simulink model "stateSpace_design_bbsim_2022"  (R2022b)
settings: Solver=ode45  StartTime=0.0  StopTime=5  RelTol=1e-3
values from neighbouring files (symbols this model uses):
  Beq = 1.9610e-06    (= 1.961e-06)    [parameters.m]
  d = 1/sqrt(2)    [parameters.m]
  deg2V = 2.5/170    (= 0.0147058823529)    [parameters.m]
  Jeq = mot.J + mld.Jh/(gbox.N)^2    [parameters.m]
  K = lqr(sysG, Q, R)    [LQR_Bryson.m]    (also in LQR_design.m; stateSpace_Integral.m = K(2:end); stateSpace_Nominal.m = acker(A,B,eig); stateSpace_design.m = K(2:end))
  Ki = 0    [LQR_Bryson.m]    (also in LQR_design.m; stateSpace_Integral.m = K(1); stateSpace_Nominal.m; stateSpace_design.m = K(1))
  Nu = N(end)    [LQR_Bryson.m]    (also in stateSpace_Integral.m; stateSpace_Nominal.m; stateSpace_design.m)
  Nx = N(1:4)    [LQR_Bryson.m]    (also in stateSpace_Integral.m; stateSpace_Nominal.m; stateSpace_design.m)
  omega_c = 2*pi*50    (= 314.159265359)    [parameters.m]
  rads2rpm = 60/2/pi    (= 9.54929658551)    [parameters.m]
  rpm2rads = 2*pi/60    (= 0.10471975512)    [parameters.m]
  V2deg = 170/2.5    (= 68)    [parameters.m]
undefined symbols (not defined in the file or in its folder): DiscIntNeverNeededParam, drv, gbox, mld, mot, sens
libraries: hdlsllib x1
settings Model: Creator=gugli  LastModifiedBy=giuliapegoraro

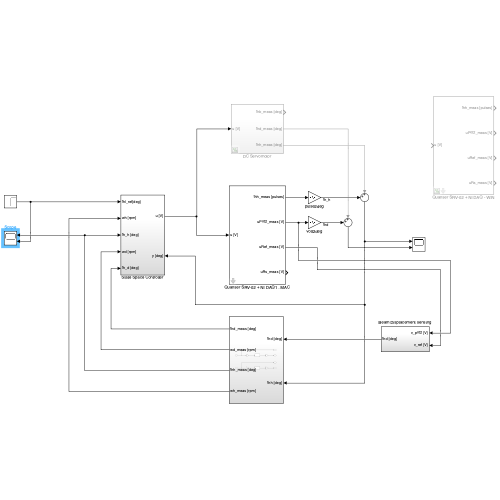
[thumbnail: Simulink's stored preview of the top-level diagram]
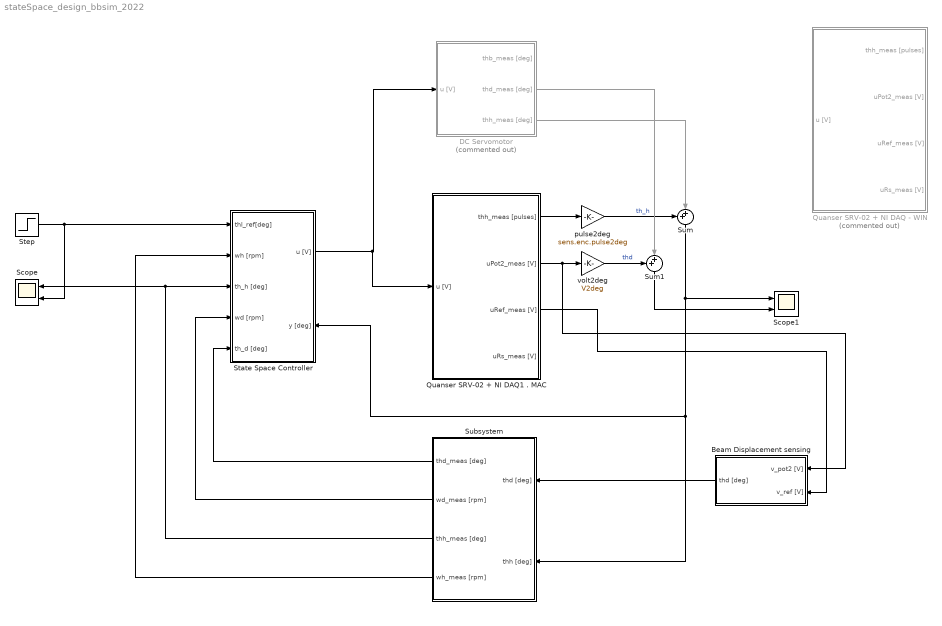
== system stateSpace_design_bbsim_2022 ==
  Beam Displacement sensing : Subsystem
  DC Servomotor : Subsystem  Commented=on
  Quanser SRV-02 + NI DAQ - WIN : Subsystem  Commented=on  mask(Quanser SRV-02 (with resonant load) + NI DAQ){Ts=0.001, fricType=Coulomb + viscous, lockShaft=off, beamInitPos=10}
      mask prompts: Ts "NI DAQ Sample Time:"; fricType "Friction model"; lockShaft "Lock motor shaft"; beamInitPos "Beam initial position [deg]:"
      mask help: Quanser SRV-02 (with resonant load) + NI DAQ model.
      mask init:
      | %%
      | % Riccardo Antonello (riccardo.antonello@unipd.it)
      | %
      | % April 28, 2020
      | %
      | % Dept. of Information Engineering, University of Padova
      | %
      | 
      | %%  Conversion gains
      | deg2rad = pi/180;                   %   [deg]   -> [rad]
      | rad2deg = 180/pi;                   %   [rad]   -> [deg]
      | 
      | 
      | %%  Sensors data
      | 
      | %   shunt resistor
      | sens.curr.Rs = 0.5;   
      | 
      | %   Hewlett-Packard HEDS-5540#A06 optical encoder
      | sens.enc.ppr = 500*4;                                                   %   pulses per rotation
      | sens.enc.pulse2deg = 360/sens.enc.ppr;                                  %   [pulses] -> [deg]
      | sens.enc.pulse2rad = 2*pi/sens.enc.ppr;                                 %   [pulses] -> [rad]
      | sens.enc.deg2pulse = sens.enc.ppr/360;                                  %   [deg] -> [pulses]
      | sens.enc.rad2pulse = sens.enc.ppr/2/pi;                                 %   [rad] -> [pulses]
      | 
      | %   potentiometer 2 (Spectrol 357-0-0-103) - installed on hub
      | sens.pot2.range.R      = 10e3;                                          %   ohmic value range 
      | sens.pot2.range.V      = 5;                                             %   voltage range
      | sens.pot2.range.th_deg = 340;                                           %   angle range [deg]
      | sens.pot2.range.th     = sens.pot2.range.th_deg * deg2rad;              %   angle range [rad]                           
      | sens.pot2.deg2V        = sens.pot2.range.V / sens.pot2.range.th_deg;    %   sensitivity [V/deg]
      | sens.pot2.rad2V        = sens.pot2.range.V / sens.pot2.range.th;        %   sensitivity [V/rad]
      | sens.pot2.V2deg        = 1/sens.pot2.deg2V;                             %   conversion gain [V] -> [deg]
      | sens.pot2.V2rad        = 1/sens.pot2.rad2V;                             %   conversion gain [V] -> [rad]
      | sens.pot2.noise.var    = 3.5e-7;                                        %   out noise variance [V^2]
      | 
      | 
      | %%  Data acquisition board (daq) data
      | 
      | %   NI PCI-6221 DAC data
      | daq.dac.bits = 16;                                  %   resolution (bits)
      | daq.dac.fs   = 10;                                  %   full scale 
      | daq.dac.q    = 2*daq.dac.fs/(2^daq.dac.bits-1);     %	quantization
      | 
      | %   NI PCI-6221 ADC data
      | daq.adc.bits = 16;                                  %   resolution (bits)
      | daq.adc.fs   = 10;                                  %   full scale (as set in SLDRT Analog Input block)
      | daq.adc.q    = 2*daq.adc.fs/(2^daq.adc.bits-1);     %   quantization   
      | 
      | 
      | %%  Set beam initial position
      | % SRV02Handle = find_system(gcb, ...
      | %     'LookUnderMasks', 'on', ...
      | %     'FindAll', 'on', ...
      | %     'FollowLinks', 'on', ...
      | %     'SearchDepth', '1', ...
      | %     'BlockType', 'ModelReference', ...
      | %     'Name', 'Quanser SRV-02');
      | %
      | % %get_param(SRV02Handle, 'InstanceParameters')
      | % InstanceParams = get_param(SRV02Handle, 'InstanceParameters');
      | % for k = 1:length(InstanceParams)
      | %     if strcmp(InstanceParams(k).Name, 'thb0')
      | %         if lockShaft
      | %             InstanceParams(k).Value = sprintf('%f', beamInitPos);
      | %         else
      | %             InstanceParams(k).Value = sprintf('%f', 0);    
      | %         end
      | %         set_param(SRV02Handle, 'InstanceParameters', InstanceParams);
      | %         break;
      | %     end
      | % end
      | 
      | if lockShaft
      |     thb0 = beamInitPos;
      | else
      |     thb0 = 0;    
      | end
      | 
      | 
      | %%  Mask initialization
      | if lockShaft
      |     
      |     %   find Inport handle
      |     InPortHandle = find_system(gcb, ...
      |         'LookUnderMasks', 'on', ...
      |         'FindAll', 'on', ...
      |         'FollowLinks', 'on', ...
      |         'SearchDepth', '1', ...
      |         'BlockType', 'Inport', ...
      |         'Name', 'u [V]');
      |     
      |     if ~isempty(InPortHandle)
      |     
      |         %   find DAC handle
      |         DACHandle = find_system(gcb, ...
      |             'LookUnderMasks', 'on', ...
      |             'FindAll', 'on', ...
      |             'FollowLinks', 'on', ...
      |             'SearchDepth', '1', ...
      |             'BlockType', 'SubSystem', ...
      |             'Name', 'DAC');  
      | 
      |         %   remove Inport output connection   
      |         InportConn = get_param(InPortHandle, 'PortConnectivity');
      |         delete_line(gcb, InportConn.Position);
      | 
      |         %   remove Inport block
      |         delete_block(InPortHandle);
      | 
      |         %   add Constant block
      |         ConstantHandle = add_block( ...
      |             'simulink/Sources/Constant', [gcb, '/u [V]'], ...
      |             'Position', [20   -37    50   -23], ...
      |             'Value', '0');
      | 
      |         %   connect Constant to DAC block
      |         DACPortHandles = get_param(DACHandle, 'PortHandles');
      |         ConstantPortHandles = get_param(ConstantHandle, 'PortHandles');
      |         add_line(gcb, ConstantPortHandles.Outport(1), DACPortHandles.Inport(1));
      |     
      |     end
      |     
      | else
      |     
      |     %   find Constant handle
      |     ConstantHandle = find_system(gcb, ...
      |         'LookUnderMasks', 'on', ...
      |         'FindAll', 'on', ...
      |         'FollowLinks', 'on', ...
      |         'SearchDepth', '1', ...
      |         'BlockType', 'Constant', ...
      |         'Name', 'u [V]');
      |     
      |     if ~isempty(ConstantHandle)
      |     
      |         %   find DAC handle
      |         DACHandle = find_system(gcb, ...
      |             'LookUnderMasks', 'on', ...
      |             'FindAll', 'on', ...
      |             'FollowLinks', 'on', ...
      |             'SearchDepth', '1', ...
      |             'BlockType', 'SubSystem', ...
      |             'Name', 'DAC');  
      |  
      |         %   remove Constant output connection   
      |         ConstantConn = get_param(ConstantHandle, 'PortConnectivity');
      |         delete_line(gcb, ConstantConn.Position);
      | 
      |         %   remove Inport block
      |         delete_block(ConstantHandle);   
      | 
      |         %   add Inport block
      |         InportHandle = add_block( ...
      |             'simulink/Sources/In1', [gcb, '/u [V]'], ...
      |             'Position', [20   -37    50   -23], ...
      |             'Port', '1');
      | 
      |         %   connect Constant to DAC block
      |         DACPortHandles = get_param(DACHandle, 'PortHandles');
      |         InportPortHandles = get_param(InportHandle, 'PortHandles');
      |         add_line(gcb, InportPortHandles.Outport(1), DACPortHandles.Inport(1));
      |     
      |      end
      |     
      | end
      mask Help:
      | Riccardo Antonello (antonello@dei.unipd.it)
      | 
      | April 28, 2020
      | 
      | Dept. of Information Engineering, University of Padova
      mask TypeOptions fricType: Coulomb + viscous | Karnopp
      mask Callback lockShaft:
      | %   get status of check box
      | lockShaft = get_param(gcb, 'lockShaft');
      | 
      | %   get current value of MaskVisibilities property
      | maskVisibilities = get_param(gcb, 'MaskVisibilities');
      | 
      | %   set visibility of the dialog box element
      | if strcmp(lockShaft, 'on')
      |     maskVisibilities{4} = 'on';
      | else
      |     maskVisibilities{4} = 'off';
      | end
      | 
      | % Set the 'MaskVisibilities' property for each parameter in mask
      | set_param( gcb, 'MaskVisibilities', maskVisibilities);
  Quanser SRV-02 + NI DAQ1 . MAC : Subsystem  mask(Quanser SRV-02 (with resonant load) + NI DAQ){Ts=0.001, fricType=Coulomb + viscous, lockShaft=off, beamInitPos=10}
      mask prompts: Ts "NI DAQ Sample Time:"; fricType "Friction model"; lockShaft "Lock motor shaft"; beamInitPos "Beam initial position [deg]:"
      mask help: Quanser SRV-02 (with resonant load) + NI DAQ model.
      mask init: same as stateSpace_design_bbsim_2022/Quanser SRV-02 + NI DAQ - WIN
      mask Help:
      | Riccardo Antonello (antonello@dei.unipd.it)
      | 
      | April 28, 2020
      | 
      | Dept. of Information Engineering, University of Padova
      mask TypeOptions fricType: Coulomb + viscous | Karnopp
      mask Callback lockShaft:
      | %   get status of check box
      | lockShaft = get_param(gcb, 'lockShaft');
      | 
      | %   get current value of MaskVisibilities property
      | maskVisibilities = get_param(gcb, 'MaskVisibilities');
      | 
      | %   set visibility of the dialog box element
      | if strcmp(lockShaft, 'on')
      |     maskVisibilities{4} = 'on';
      | else
      |     maskVisibilities{4} = 'off';
      | end
      | 
      | % Set the 'MaskVisibilities' property for each parameter in mask
      | set_param( gcb, 'MaskVisibilities', maskVisibilities);
  Scope : Scope  NumInputPorts=2
  Scope1 : Scope  NumInputPorts=2
  State Space Controller : Subsystem
      settings: PortSchema="{\"entries\":[{\"content\":{\"sides\":[{\"content\":{\"connectorIds\":[\"In1\",\"In2\",\"In3\",\"In4\",\"In5\"]},\"type\":\"ConnectorPlacement.EquallySpacedRectSide\",\"uuid\":\"18355374-ba4e-4826-b39c-e1fec12a3224\"},{\"content\":{\"connectorIds\":[\"Out1\",\"In6\"],\"side\":\"RIGHT\"},\"type\":\"ConnectorPlacement.EquallySpacedRectSide\",\"uuid\":\"1b1017b5-1e71-4f75-9751-b5be90c6ae70\"},{\"content\":{\"connectorIds\":[],\"side\":\"TOP\"},\"type\":\"ConnectorPlacement.EquallySpacedRectSide\",\"uuid\":\"216eee75-1744-4a6a-833a-20d97cc02b89\"}]},\"type\":\"ConnectorPlacement.EquallySpacedConnector\",\"uuid\":\"af6359b3-3eb7-4cad-ada4-005509c30a45\"}],\"packageUris\":[\"http://schema.mathworks.com/mf0/Connector/R2020b\"],\"version\":\"1.0\"}"
  Step : Step  After=50
  Subsystem : Subsystem
  Sum : Sum  Inputs=++|
  Sum1 : Sum  Inputs=++|
  pulse2deg : Gain  Gain=sens.enc.pulse2deg
  volt2deg : Gain  Gain=V2deg
  wires:
  Step/1 -> Scope/2, State Space Controller/1(thl_ref[deg])
  pulse2deg/1 -> Sum/1  "th_h"
  DC Servomotor/3(thh_meas [deg]) -> Sum/2
  Quanser SRV-02 + NI DAQ1 . MAC/1(thh_meas [pulses]) -> pulse2deg/1
  State Space Controller/1(u [V]) -> Quanser SRV-02 + NI DAQ1 . MAC/1(u [V]), DC Servomotor/1(u [V])
  Quanser SRV-02 + NI DAQ1 . MAC/2(uPot2_meas [V]) -> Beam Displacement sensing/1(v_pot2 [V]), volt2deg/1
  Subsystem/1(thd_meas [deg]) -> State Space Controller/5(th_d [deg])
  Subsystem/2(wd_meas [rpm]) -> State Space Controller/4(wd [rpm])
  Subsystem/3(thh_meas [deg]) -> Scope/1, State Space Controller/3(th_h [deg])
  Subsystem/4(wh_meas [rpm]) -> State Space Controller/2(wh [rpm])
  Sum1/1 -> Scope1/2
  volt2deg/1 -> Sum1/1  "thd"
  DC Servomotor/2(thd_meas [deg]) -> Sum1/2
  Sum/1 -> State Space Controller/6(y [deg]), Subsystem/2(thh [deg]), Scope1/1
  Quanser SRV-02 + NI DAQ1 . MAC/3(uRef_meas [V]) -> Beam Displacement sensing/2(v_ref [V])
  Beam Displacement sensing/1(thd [deg]) -> Subsystem/1(thd [deg])

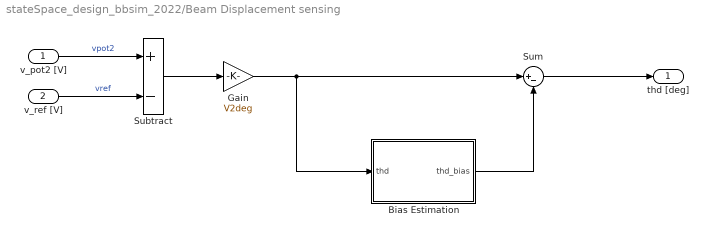
== system stateSpace_design_bbsim_2022/Beam Displacement sensing ==
  v_pot2 [V] : Inport
  v_ref [V] : Inport  Port=2
  Bias Estimation : Subsystem
  Gain : Gain  Gain=V2deg
  Subtract : Sum  Inputs=+-
  Sum : Sum  Inputs=|+-
  thd [deg] : Outport
  wires:
  v_ref [V]/1 -> Subtract/2  "vref"
  v_pot2 [V]/1 -> Subtract/1  "vpot2"
  Subtract/1 -> Gain/1
  Gain/1 -> Bias Estimation/1(thd), Sum/1
  Sum/1 -> thd [deg]/1
  Bias Estimation/1(thd_bias) -> Sum/2

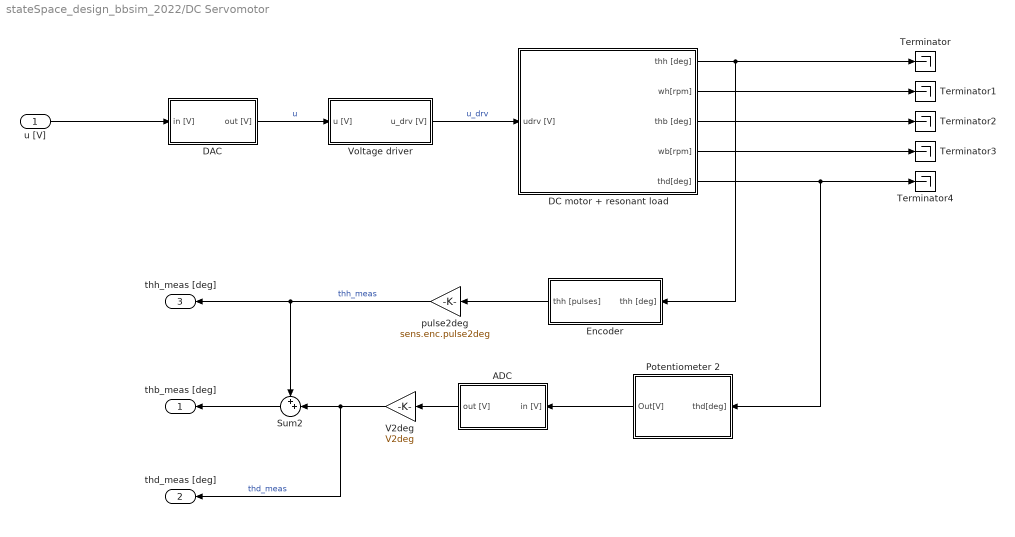
== system stateSpace_design_bbsim_2022/DC Servomotor ==
  u [V] : Inport
  ADC : Subsystem
  DAC : Subsystem
  DC motor + resonant load : Subsystem
  Encoder : Subsystem
  Potentiometer 2 : Subsystem
  Sum2 : Sum  Inputs=++|
  Terminator{,1..4} (5 alike) : Terminator
  V2deg : Gain  Gain=V2deg
  Voltage driver : Subsystem
  pulse2deg : Gain  Gain=sens.enc.pulse2deg
  thb_meas [deg] : Outport
  thd_meas [deg] : Outport  Port=2
  thh_meas [deg] : Outport  Port=3
  wires:
  Encoder/1(thh [pulses]) -> pulse2deg/1
  DAC/1(out [V]) -> Voltage driver/1(u [V])  "u"
  pulse2deg/1 -> thh_meas [deg]/1, Sum2/1  "thh_meas"
  u [V]/1 -> DAC/1(in [V])
  DC motor + resonant load/1(thh [deg]) -> Encoder/1(thh [deg]), Terminator/1
  DC motor + resonant load/2(wh[rpm]) -> Terminator1/1
  Voltage driver/1(u_drv [V]) -> DC motor + resonant load/1(udrv [V])  "u_drv"
  DC motor + resonant load/3(thb [deg]) -> Terminator2/1
  DC motor + resonant load/4(wb[rpm]) -> Terminator3/1
  DC motor + resonant load/5(thd[deg]) -> Potentiometer 2/1(thd[deg]), Terminator4/1
  Potentiometer 2/1(Out[V]) -> ADC/1(in [V])
  ADC/1(out [V]) -> V2deg/1
  V2deg/1 -> thd_meas [deg]/1, Sum2/2  "thd_meas"
  Sum2/1 -> thb_meas [deg]/1

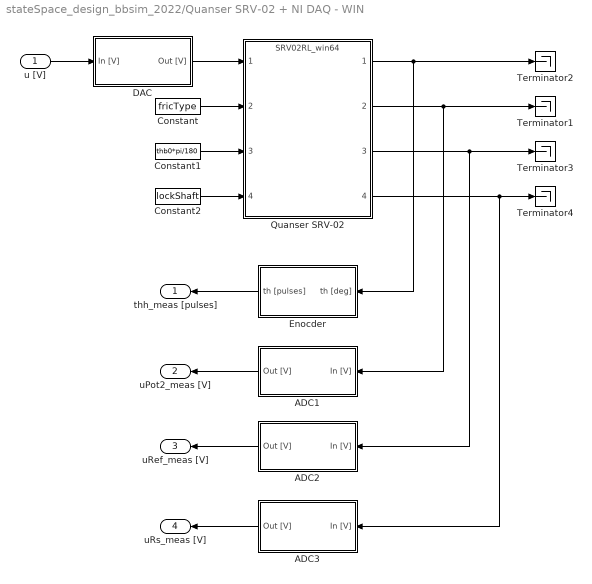
== system stateSpace_design_bbsim_2022/Quanser SRV-02 + NI DAQ - WIN ==
  u [V] : Inport
  ADC1 : Subsystem
  ADC2 : Subsystem
  ADC3 : Subsystem
  Constant : Constant  Value=fricType
  Constant1 : Constant  Value=thb0*pi/180  SampleTime=Inf
  Constant2 : Constant  Value=lockShaft  SampleTime=Inf
  DAC : Subsystem
  Enocder : Subsystem
  Quanser SRV-02 : ModelReference  ModelNameDialog=SRV02RL_win64.slxp  ModelReferenceVersion=1.76  CopyOfModelProtected=on
  Terminator{1..4} (4 alike) : Terminator
  thh_meas [pulses] : Outport
  uPot2_meas [V] : Outport  Port=2
  uRef_meas [V] : Outport  Port=3
  uRs_meas [V] : Outport  Port=4
  wires:
  u [V]/1 -> DAC/1(In [V])
  ADC2/1(Out [V]) -> uRef_meas [V]/1
  Quanser SRV-02/4 -> Terminator4/1, ADC3/1(In [V])
  Constant2/1 -> Quanser SRV-02/4
  Constant1/1 -> Quanser SRV-02/3
  ADC1/1(Out [V]) -> uPot2_meas [V]/1
  Quanser SRV-02/3 -> Terminator3/1, ADC2/1(In [V])
  Constant/1 -> Quanser SRV-02/2
  Quanser SRV-02/1 -> Enocder/1(th [deg]), Terminator2/1
  Quanser SRV-02/2 -> Terminator1/1, ADC1/1(In [V])
  DAC/1(Out [V]) -> Quanser SRV-02/1
  ADC3/1(Out [V]) -> uRs_meas [V]/1
  Enocder/1(th [pulses]) -> thh_meas [pulses]/1

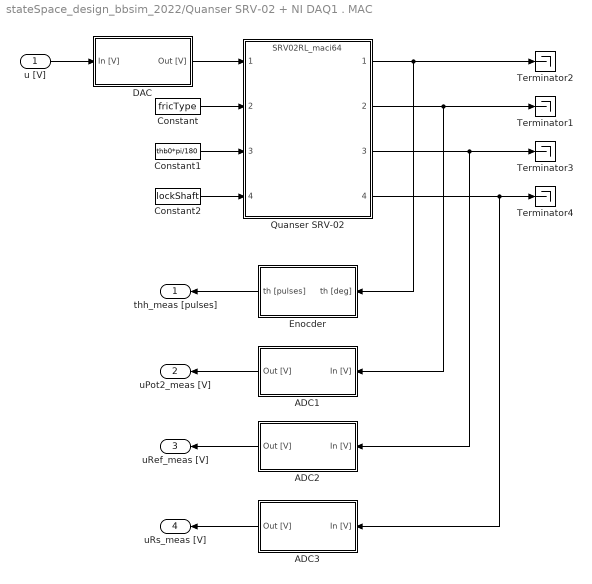
== system stateSpace_design_bbsim_2022/Quanser SRV-02 + NI DAQ1 . MAC ==
  u [V] : Inport
  ADC1 : Subsystem
  ADC2 : Subsystem
  ADC3 : Subsystem
  Constant : Constant  Value=fricType
  Constant1 : Constant  Value=thb0*pi/180  SampleTime=Inf
  Constant2 : Constant  Value=lockShaft  SampleTime=Inf
  DAC : Subsystem
  Enocder : Subsystem
  Quanser SRV-02 : ModelReference  ModelNameDialog=SRV02RL_maci64.slxp  ModelReferenceVersion=1.76  CopyOfModelProtected=on
  Terminator{1..4} (4 alike) : Terminator
  thh_meas [pulses] : Outport
  uPot2_meas [V] : Outport  Port=2
  uRef_meas [V] : Outport  Port=3
  uRs_meas [V] : Outport  Port=4
  wires:
  Enocder/1(th [pulses]) -> thh_meas [pulses]/1
  ADC3/1(Out [V]) -> uRs_meas [V]/1
  DAC/1(Out [V]) -> Quanser SRV-02/1
  Quanser SRV-02/2 -> ADC1/1(In [V]), Terminator1/1
  Quanser SRV-02/1 -> Terminator2/1, Enocder/1(th [deg])
  Constant/1 -> Quanser SRV-02/2
  Quanser SRV-02/3 -> ADC2/1(In [V]), Terminator3/1
  ADC1/1(Out [V]) -> uPot2_meas [V]/1
  Constant1/1 -> Quanser SRV-02/3
  Constant2/1 -> Quanser SRV-02/4
  u [V]/1 -> DAC/1(In [V])
  Quanser SRV-02/4 -> ADC3/1(In [V]), Terminator4/1
  ADC2/1(Out [V]) -> uRef_meas [V]/1

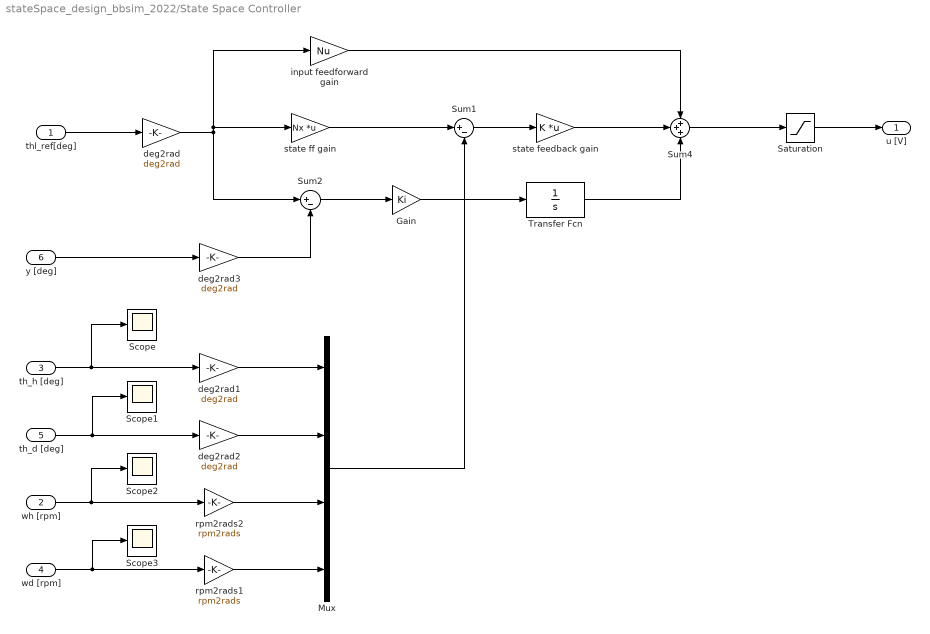
== system stateSpace_design_bbsim_2022/State Space Controller ==
  thl_ref[deg] : Inport
  wh [rpm] : Inport  Port=2
  th_h [deg] : Inport  Port=3
  wd [rpm] : Inport  Port=4
  th_d [deg] : Inport  Port=5
  y [deg] : Inport  Port=6
  " Saturation" : Saturate  UpperLimit=12  LowerLimit=-12
  Gain : Gain  Gain=Ki
  Mux : Mux
  Scope{,1..3} (4 alike) : Scope
  Sum1 : Sum  Inputs=|+-
  Sum2 : Sum  Inputs=|+-
  Sum4 : Sum  Inputs=+++
  Transfer Fcn : TransferFcn  Numerator=1  Denominator=[1 0]
  deg2rad{,1..3} (4 alike) : Gain  Gain=deg2rad
  input feedforward gain : Gain  Gain=Nu
  rpm2rads1 : Gain  Gain=rpm2rads
  rpm2rads2 : Gain  Gain=rpm2rads
  state feedback gain : Gain  Gain=K  Multiplication=Matrix(K*u) (u vector)
  state ff gain : Gain  Gain=Nx  Multiplication=Matrix(K*u) (u vector)
  u [V] : Outport
  wires:
  thl_ref[deg]/1 -> deg2rad/1
  deg2rad/1 -> state ff gain/1, input feedforward gain/1, Sum2/1
  state ff gain/1 -> Sum1/1
  Sum1/1 -> state feedback gain/1
  state feedback gain/1 -> Sum4/2
  input feedforward gain/1 -> Sum4/1
  Sum4/1 -> " Saturation"/1
  " Saturation"/1 -> u [V]/1
  Mux/1 -> Sum1/2
  deg2rad1/1 -> Mux/1
  th_h [deg]/1 -> Scope/1, deg2rad1/1
  wd [rpm]/1 -> Scope3/1, rpm2rads1/1
  rpm2rads1/1 -> Mux/4
  Gain/1 -> Transfer Fcn/1
  Transfer Fcn/1 -> Sum4/3
  y [deg]/1 -> deg2rad3/1
  deg2rad3/1 -> Sum2/2
  Sum2/1 -> Gain/1
  rpm2rads2/1 -> Mux/3
  deg2rad2/1 -> Mux/2
  th_d [deg]/1 -> Scope1/1, deg2rad2/1
  wh [rpm]/1 -> Scope2/1, rpm2rads2/1

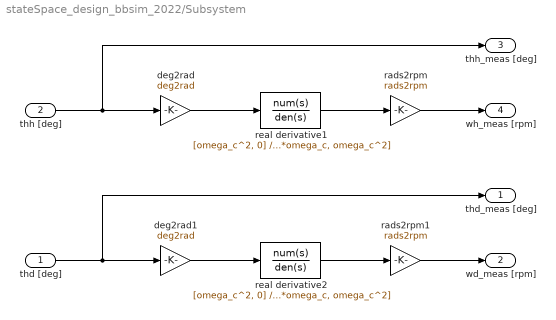
== system stateSpace_design_bbsim_2022/Subsystem ==
  thd [deg] : Inport
  thh [deg] : Inport  Port=2
  deg2rad : Gain  Gain=deg2rad
  deg2rad1 : Gain  Gain=deg2rad
  rads2rpm : Gain  Gain=rads2rpm
  rads2rpm1 : Gain  Gain=rads2rpm
  real derivative1 : TransferFcn  Numerator=[omega_c^2, 0]  Denominator=[1, 2*d*omega_c, omega_c^2]
  real derivative2 : TransferFcn  Numerator=[omega_c^2, 0]  Denominator=[1, 2*d*omega_c, omega_c^2]
  thd_meas [deg] : Outport
  wd_meas [rpm] : Outport  Port=2
  thh_meas [deg] : Outport  Port=3
  wh_meas [rpm] : Outport  Port=4
  wires:
  deg2rad/1 -> real derivative1/1
  thh [deg]/1 -> thh_meas [deg]/1, deg2rad/1
  real derivative1/1 -> rads2rpm/1
  rads2rpm/1 -> wh_meas [rpm]/1
  rads2rpm1/1 -> wd_meas [rpm]/1
  thd [deg]/1 -> thd_meas [deg]/1, deg2rad1/1
  deg2rad1/1 -> real derivative2/1
  real derivative2/1 -> rads2rpm1/1

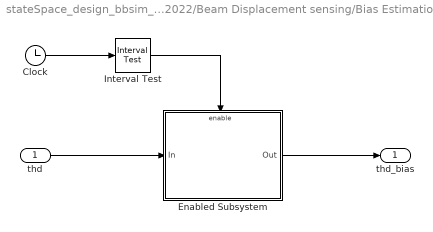
== system stateSpace_design_bbsim_2022/Beam Displacement sensing/Bias Estimation ==
  thd : Inport
  Clock : Clock
  Enabled Subsystem : Subsystem  TreatAsAtomicUnit=on
  Interval Test : hdlsllib/Logic and Bit Operations/Interval Test  IntervalClosedRight=on  uplimit=0.5  IntervalClosedLeft=on  lowlimit=-0.5  OutDataTypeStr=boolean
  thd_bias : Outport
  wires:
  thd/1 -> Enabled Subsystem/1(In)
  Enabled Subsystem/1(Out) -> thd_bias/1
  Clock/1 -> Interval Test/1
  Interval Test/1 -> Enabled Subsystem/Enable

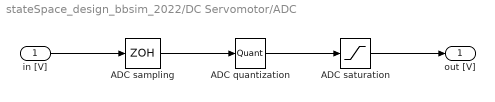
== system stateSpace_design_bbsim_2022/DC Servomotor/ADC ==
  in [V] : Inport
  ADC quantization : Quantizer  QuantizationInterval=daq.adc.q
  ADC sampling : ZeroOrderHold  SampleTime=0.001
  ADC saturation : Saturate  UpperLimit=10  LowerLimit=-10
  out [V] : Outport
  wires:
  ADC saturation/1 -> out [V]/1
  ADC quantization/1 -> ADC saturation/1
  in [V]/1 -> ADC sampling/1
  ADC sampling/1 -> ADC quantization/1

== system stateSpace_design_bbsim_2022/DC Servomotor/DAC ==
  in [V] : Inport
  Quantizer : Quantizer  QuantizationInterval=daq.dac.q
  Saturation : Saturate  UpperLimit=10  LowerLimit=-10
  Zero-Order Hold : ZeroOrderHold  SampleTime=0.001
  out [V] : Outport
  wires:
  Saturation/1 -> out [V]/1
  Quantizer/1 -> Saturation/1
  in [V]/1 -> Zero-Order Hold/1
  Zero-Order Hold/1 -> Quantizer/1

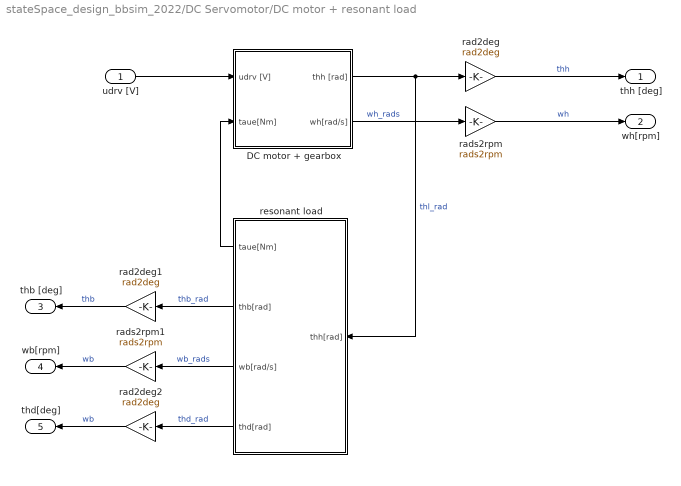
== system stateSpace_design_bbsim_2022/DC Servomotor/DC motor + resonant load ==
  udrv [V] : Inport
  DC motor + gearbox : Subsystem
  rad2deg : Gain  Gain=rad2deg
  rad2deg1 : Gain  Gain=rad2deg
  rad2deg2 : Gain  Gain=rad2deg
  rads2rpm : Gain  Gain=rads2rpm
  rads2rpm1 : Gain  Gain=rads2rpm
  resonant load : Subsystem
  thh [deg] : Outport
  wh[rpm] : Outport  Port=2
  thb [deg] : Outport  Port=3
  wb[rpm] : Outport  Port=4
  thd[deg] : Outport  Port=5
  wires:
  DC motor + gearbox/1(thh [rad]) -> resonant load/1(thh[rad]), rad2deg/1  "thl_rad"
  rad2deg2/1 -> thd[deg]/1  "wb"
  resonant load/1(taue[Nm]) -> DC motor + gearbox/2(taue[Nm])
  DC motor + gearbox/2(wh[rad/s]) -> rads2rpm/1  "wh_rads"
  rad2deg/1 -> thh [deg]/1  "thh"
  resonant load/4(thd[rad]) -> rad2deg2/1  "thd_rad"
  rads2rpm/1 -> wh[rpm]/1  "wh"
  udrv [V]/1 -> DC motor + gearbox/1(udrv [V])
  resonant load/2(thb[rad]) -> rad2deg1/1  "thb_rad"
  resonant load/3(wb[rad/s]) -> rads2rpm1/1  "wb_rads"
  rads2rpm1/1 -> wb[rpm]/1  "wb"
  rad2deg1/1 -> thb [deg]/1  "thb"

== system stateSpace_design_bbsim_2022/DC Servomotor/Encoder ==
  thh [deg] : Inport
  Gain : Gain  Gain=1/sens.enc.pulse2deg
  Quantizer : Quantizer  QuantizationInterval=sens.enc.pulse2deg
  Zero-Order Hold : ZeroOrderHold  SampleTime=0.001
  thh [pulses] : Outport
  wires:
  Zero-Order Hold/1 -> Quantizer/1
  thh [deg]/1 -> Zero-Order Hold/1
  Quantizer/1 -> Gain/1
  Gain/1 -> thh [pulses]/1

== system stateSpace_design_bbsim_2022/DC Servomotor/Potentiometer 2 ==
  thd[deg] : Inport
  Sum2 : Sum  Inputs=++|
  deg2V : Gain  Gain=deg2V
  sensor output noise [V] : RandomNumber  Variance=3.5*10^[-7]  SampleTime=0.001
  Out[V] : Outport
  wires:
  Sum2/1 -> Out[V]/1
  sensor output noise [V]/1 -> Sum2/1
  deg2V/1 -> Sum2/2  "thl_meas"
  thd[deg]/1 -> deg2V/1

== system stateSpace_design_bbsim_2022/DC Servomotor/Voltage driver ==
  u [V] : Inport
  Saturation : Saturate  UpperLimit=12  LowerLimit=-12
  Transfer Fcn : TransferFcn  Numerator=[drv.dcgain]  Denominator=[drv.Tc 1]
  u_drv [V] : Outport
  wires:
  Saturation/1 -> u_drv [V]/1
  Transfer Fcn/1 -> Saturation/1
  u [V]/1 -> Transfer Fcn/1

== system stateSpace_design_bbsim_2022/Quanser SRV-02 + NI DAQ - WIN/ADC1 ==
  In [V] : Inport
  ADC quantization : Quantizer  QuantizationInterval=daq.adc.q
  ADC sampling : ZeroOrderHold  SampleTime=Ts
  ADC saturation : Saturate  UpperLimit=daq.adc.fs  LowerLimit=-daq.adc.fs
  Out [V] : Outport
  wires:
  ADC quantization/1 -> ADC saturation/1
  In [V]/1 -> ADC sampling/1
  ADC sampling/1 -> ADC quantization/1
  ADC saturation/1 -> Out [V]/1

== system stateSpace_design_bbsim_2022/Quanser SRV-02 + NI DAQ - WIN/ADC2 ==
  In [V] : Inport
  ADC quantization : Quantizer  QuantizationInterval=daq.adc.q
  ADC sampling : ZeroOrderHold  SampleTime=Ts
  ADC saturation : Saturate  UpperLimit=daq.adc.fs  LowerLimit=-daq.adc.fs
  Out [V] : Outport
  wires:
  ADC saturation/1 -> Out [V]/1
  ADC sampling/1 -> ADC quantization/1
  In [V]/1 -> ADC sampling/1
  ADC quantization/1 -> ADC saturation/1

== system stateSpace_design_bbsim_2022/Quanser SRV-02 + NI DAQ - WIN/ADC3 ==
  In [V] : Inport
  Quantizer : Quantizer  QuantizationInterval=daq.adc.q
  Saturation : Saturate  UpperLimit=daq.adc.fs  LowerLimit=-daq.adc.fs
  Zero-Order Hold : ZeroOrderHold  SampleTime=Ts
  Out [V] : Outport
  wires:
  Zero-Order Hold/1 -> Quantizer/1
  Quantizer/1 -> Saturation/1
  In [V]/1 -> Zero-Order Hold/1
  Saturation/1 -> Out [V]/1

== system stateSpace_design_bbsim_2022/Quanser SRV-02 + NI DAQ - WIN/DAC ==
  In [V] : Inport
  Quantizer : Quantizer  QuantizationInterval=daq.dac.q
  Saturation : Saturate  UpperLimit=daq.dac.fs  LowerLimit=-daq.dac.fs
  Zero-Order Hold : ZeroOrderHold  SampleTime=Ts
  Out [V] : Outport
  wires:
  Saturation/1 -> Out [V]/1
  Zero-Order Hold/1 -> Quantizer/1
  In [V]/1 -> Zero-Order Hold/1
  Quantizer/1 -> Saturation/1

== system stateSpace_design_bbsim_2022/Quanser SRV-02 + NI DAQ - WIN/Enocder ==
  th [deg] : Inport
  Quantizer : Quantizer  QuantizationInterval=sens.enc.pulse2deg
  Zero-Order Hold : ZeroOrderHold  SampleTime=Ts
  deg2pulse : Gain  Gain=sens.enc.deg2pulse
  th [pulses] : Outport
  wires:
  deg2pulse/1 -> th [pulses]/1
  Zero-Order Hold/1 -> Quantizer/1
  th [deg]/1 -> Zero-Order Hold/1
  Quantizer/1 -> deg2pulse/1

== system stateSpace_design_bbsim_2022/Quanser SRV-02 + NI DAQ1 . MAC/ADC1 ==
  In [V] : Inport
  ADC quantization : Quantizer  QuantizationInterval=daq.adc.q
  ADC sampling : ZeroOrderHold  SampleTime=Ts
  ADC saturation : Saturate  UpperLimit=daq.adc.fs  LowerLimit=-daq.adc.fs
  Out [V] : Outport
  wires:
  ADC saturation/1 -> Out [V]/1
  ADC sampling/1 -> ADC quantization/1
  In [V]/1 -> ADC sampling/1
  ADC quantization/1 -> ADC saturation/1

== system stateSpace_design_bbsim_2022/Quanser SRV-02 + NI DAQ1 . MAC/ADC2 ==
  In [V] : Inport
  ADC quantization : Quantizer  QuantizationInterval=daq.adc.q
  ADC sampling : ZeroOrderHold  SampleTime=Ts
  ADC saturation : Saturate  UpperLimit=daq.adc.fs  LowerLimit=-daq.adc.fs
  Out [V] : Outport
  wires:
  ADC quantization/1 -> ADC saturation/1
  In [V]/1 -> ADC sampling/1
  ADC sampling/1 -> ADC quantization/1
  ADC saturation/1 -> Out [V]/1

== system stateSpace_design_bbsim_2022/Quanser SRV-02 + NI DAQ1 . MAC/ADC3 ==
  In [V] : Inport
  Quantizer : Quantizer  QuantizationInterval=daq.adc.q
  Saturation : Saturate  UpperLimit=daq.adc.fs  LowerLimit=-daq.adc.fs
  Zero-Order Hold : ZeroOrderHold  SampleTime=Ts
  Out [V] : Outport
  wires:
  Saturation/1 -> Out [V]/1
  In [V]/1 -> Zero-Order Hold/1
  Quantizer/1 -> Saturation/1
  Zero-Order Hold/1 -> Quantizer/1

== system stateSpace_design_bbsim_2022/Quanser SRV-02 + NI DAQ1 . MAC/DAC ==
  In [V] : Inport
  Quantizer : Quantizer  QuantizationInterval=daq.dac.q
  Saturation : Saturate  UpperLimit=daq.dac.fs  LowerLimit=-daq.dac.fs
  Zero-Order Hold : ZeroOrderHold  SampleTime=Ts
  Out [V] : Outport
  wires:
  Quantizer/1 -> Saturation/1
  In [V]/1 -> Zero-Order Hold/1
  Zero-Order Hold/1 -> Quantizer/1
  Saturation/1 -> Out [V]/1

== system stateSpace_design_bbsim_2022/Quanser SRV-02 + NI DAQ1 . MAC/Enocder ==
  th [deg] : Inport
  Quantizer : Quantizer  QuantizationInterval=sens.enc.pulse2deg
  Zero-Order Hold : ZeroOrderHold  SampleTime=Ts
  deg2pulse : Gain  Gain=sens.enc.deg2pulse
  th [pulses] : Outport
  wires:
  Quantizer/1 -> deg2pulse/1
  th [deg]/1 -> Zero-Order Hold/1
  Zero-Order Hold/1 -> Quantizer/1
  deg2pulse/1 -> th [pulses]/1

== system stateSpace_design_bbsim_2022/Beam Displacement sensing/Bias Estimation/Enabled Subsystem ==
  In : Inport
  Enable : EnablePort
  Discrete-Time Integrator : DiscreteIntegrator  SampleTime=-1  ICPrevOutput=DiscIntNeverNeededParam  ICPrevScaledInput=DiscIntNeverNeededParam
  Out : Outport
  wires:
  In/1 -> Discrete-Time Integrator/1
  Discrete-Time Integrator/1 -> Out/1

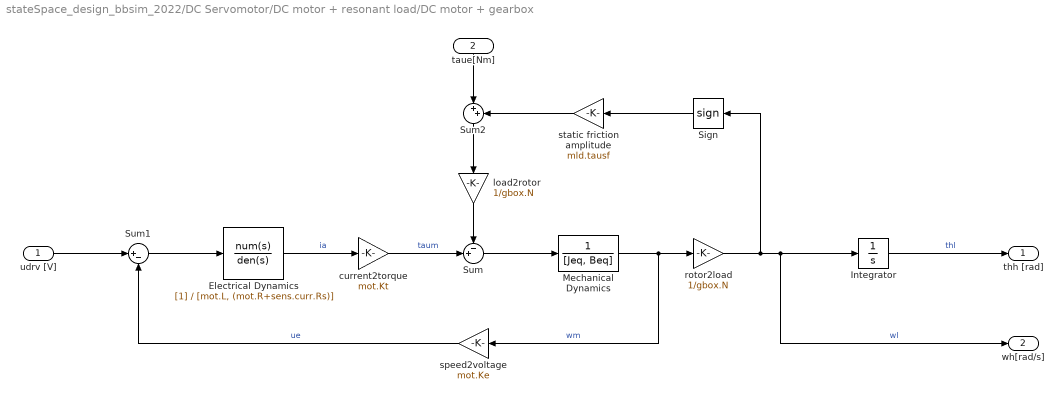
== system stateSpace_design_bbsim_2022/DC Servomotor/DC motor + resonant load/DC motor + gearbox ==
  udrv [V] : Inport
  taue[Nm] : Inport  Port=2
  Electrical Dynamics : TransferFcn  Denominator=[mot.L, (mot.R+sens.curr.Rs)]
  Integrator : Integrator
  Mechanical Dynamics : TransferFcn  Denominator=[Jeq, Beq]
  Sign : Signum  ZeroCross=off
  Sum : Sum  Inputs=-+|
  Sum1 : Sum  Inputs=|+-
  Sum2 : Sum  Inputs=|++
  current2torque : Gain  Gain=mot.Kt
  load2rotor : Gain  Gain=1/gbox.N
  rotor2load : Gain  Gain=1/gbox.N
  speed2voltage : Gain  Gain=mot.Ke
  static friction amplitude : Gain  Gain=mld.tausf
  thh [rad] : Outport
  wh[rad/s] : Outport  Port=2
  wires:
  udrv [V]/1 -> Sum1/1
  load2rotor/1 -> Sum/1
  Sign/1 -> static friction amplitude/1
  Electrical Dynamics/1 -> current2torque/1  "ia"
  current2torque/1 -> Sum/2  "taum"
  speed2voltage/1 -> Sum1/2  "ue"
  Mechanical Dynamics/1 -> rotor2load/1, speed2voltage/1  "wm"
  Integrator/1 -> thh [rad]/1  "thl"
  Sum1/1 -> Electrical Dynamics/1
  rotor2load/1 -> wh[rad/s]/1, Integrator/1, Sign/1  "wl"
  Sum/1 -> Mechanical Dynamics/1
  static friction amplitude/1 -> Sum2/2
  Sum2/1 -> load2rotor/1
  taue[Nm]/1 -> Sum2/1

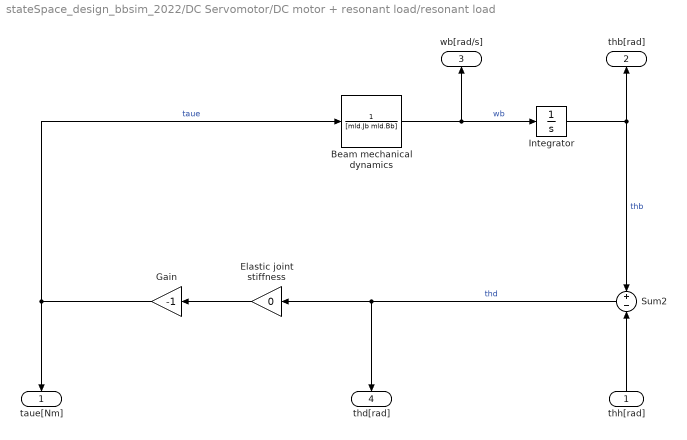
== system stateSpace_design_bbsim_2022/DC Servomotor/DC motor + resonant load/resonant load ==
  thh[rad] : Inport
  Beam mechanical dynamics : TransferFcn  Numerator=1  Denominator=[mld.Jb mld.Bb]
  Elastic joint stiffness : Gain  Gain=0
  Gain : Gain  Gain=-1
  Integrator : Integrator
  Sum2 : Sum  Inputs=+-
  taue[Nm] : Outport
  thb[rad] : Outport  Port=2
  wb[rad/s] : Outport  Port=3
  thd[rad] : Outport  Port=4
  wires:
  Gain/1 -> taue[Nm]/1, Beam mechanical dynamics/1  "taue"
  Elastic joint stiffness/1 -> Gain/1
  Sum2/1 -> thd[rad]/1, Elastic joint stiffness/1  "thd"
  thh[rad]/1 -> Sum2/2
  Integrator/1 -> Sum2/1, thb[rad]/1  "thb"
  Beam mechanical dynamics/1 -> wb[rad/s]/1, Integrator/1  "wb"
